simulink model "EV_thermal_charger_2015a_jmaab_Can01"  (R2015a)
settings: Solver=ode3  StartTime=0.0  StopTime=1800  FixedStep=sampling_time  RelTol=1e-3
PreLoadFcn:
  | %run('init_setting.m')
PostLoadFcn:
  | %set_param(gcs, 'SimulationCommand', 'update');
  | %load('save_param/save_P_Charger', 'P_Charger');
  | %load('save_param/save_T_User_set_temp_degC','T_User_set_temp_degC');
  | %load('save_param/save_ENV_PNT_PTTH_Temp_add_degC','ENV_PNT_PTTH_Temp_add_degC');
  | %load('save_param/save_ENV_PNT_CABIN_Temp_add_degC','ENV_PNT_CABIN_Temp_add_degC');
  | %load('save_param/save_ENV_PNT_PHI_Sunlight_W','ENV_PNT_PHI_Sunlight_W');
  | %load('save_param/save_ENV_PNT_Outside_Temp_ini_degC','ENV_PNT_Outside_Temp_ini_degC');
undefined symbols (not defined in the file or in its folder): BK_PNT_Pow_UL, BK_PNT_ReGene_vel_limit_DN_kmph, BK_PNT_ReGene_vel_limit_UP_kmph, BK_PNT_Tau_brake, Brk_LL, Brk_PGain, Brk_UL, BT_PNT_Hi_C_pol_hi_batt, BT_PNT_Hi_Capa_hi_batt_F, BT_PNT_Hi_ocv_SOC_hi_batt_OCV_V_table, BT_PNT_Hi_ocv_SOC_hi_batt_OCV_V_table_x_SOC, BT_PNT_Hi_R_hi_batt_cell, BT_PNT_Hi_R_pol_hi_batt, BT_PNT_Hi_SOC_MAX_hi_batt, BT_PNT_Hi_SOC_MIN_hi_batt, BT_PNT_Hi_SOC_START_hi_batt, BT_PNT_Lo_Capa_lo_batt_F, BT_PNT_Lo_ocv_SOC_lo_batt_OCV_V_table, BT_PNT_Lo_ocv_SOC_lo_batt_OCV_V_table_x_SOC, BT_PNT_Lo_R_lo_batt_ohm, BT_PNT_Lo_SOC_MAX_lo_batt, BT_PNT_Lo_SOC_MIN_lo_batt, BT_PNT_Lo_SOC_START_lo_batt, BTTH_CNT_P_BT_Heater_W, BTTH_CNT_P_BT_Heater_W_x_BTCells_degC, BTTH_CNT_Voltage_BTFan_V, BTTH_CNT_Voltage_BTFan_V_x_BTCells_degC, BTTH_PNT_BT_Heat_Resi_KpW, BTTH_PNT_BT_Heat_Resi_KpW_x_Wind_m3ps, BTTH_PNT_BT_Heater2BTCells_Heat_Resi_KpW, BTTH_PNT_BT_Heater_Heat_Capa_JpK, BTTH_PNT_BTBlock2BTAir_Heat_Resi_KpW, BTTH_PNT_BTBlock_Heat_Capa_JpK, BTTH_PNT_BTCells2BTBlock_Heat_Resi_KpW, BTTH_PNT_BTCells_Heat_Capa_JpK, BTTH_PNT_v_BTFan_Wind_vel_mps, BTTH_PNT_v_BTFan_Wind_vel_mps_x_V_BTFan, CATH_CNT_P_Aircon_W_LL, CATH_CNT_P_Aircon_W_UL, CATH_CNT_P_Gain_Aircon, CATH_CNT_P_Gain_PTC_Heater, CATH_CNT_P_Gain_SeatHT, CATH_CNT_P_PTC_Heater, CATH_CNT_P_PTC_Heater_W_LL, CATH_CNT_P_PTC_Heater_W_UL, CATH_CNT_P_PTC_Heater_x_T_Outside_temp_degC, CATH_CNT_P_SeatHT_W_LL, CATH_CNT_P_SeatHT_W_UL, CATH_CNT_PGain_Temp_blowout, CATH_CNT_T_Aircon_Indoor_degC, CATH_CNT_T_Aircon_Indoor_degC_x_T_blowout_degC, CATH_CNT_T_PTC_Heater_degC_UL, CATH_CNT_T_SeatHT_Temp_degC, CATH_CNT_T_SeatHT_Temp_degC_x_T_blowout_degC, CATH_CNT_V_HVAC_Fan, CATH_CNT_V_HVAC_Fan_x_T_blowout_degC, CATH_CNT_V_RDFan_V, CATH_CNT_V_RDFan_x_P_Aircon_W, CATH_PNT_Air_Convection_Heat_Resi_KpW, CATH_PNT_Air_Convection_Heat_Resi_x_mps ... (+141)
undefined symbols (not defined in the file): ACC_D_Gain, ACC_I_Gain, ACC_P_Gain
libraries: METI_Lib_vehicle_model x52, simulink x35
(part 6 of 6)

== system EV_thermal_charger_2015a_jmaab_Can01/Vehicle/CNT/VCU_CNT/VCU_CNT/trq_MG2_tgtCalc2/回転数上限超過時トルク制限処理 ==
  trq_MG2_tgt : Inport
  w_ROT_motor : Inport  Port=2
  User_Power_req : Inport  Port=3
  Compare To Zero : simulink/Logic and Bit Operations/Compare To Zero  relop=>  OutDataTypeStr=boolean
  Divide_0wari : METI_Lib_vehicle_model/Divide_0wari
  Product : Product
  Subtract2 : Sum  Inputs=+-
  Subtract3 : Sum
  radps2rpm2 : Gain  Gain=radps2rpm
  w_mot_limit : Constant  Value=VCU_CNT_w_mot_limit_rpm
  w_mot_limit1 : Constant  Value=VCU_CNT_w_mot_limit_gain
  flag_overrev : Outport
  trq_MG2_guarded : Outport  Port=2
  wires:
  w_ROT_motor/1 -> radps2rpm2/1
  w_mot_limit/1 -> Subtract2/1
  Subtract2/1 -> Product/1, Compare To Zero/1
  Subtract3/1 -> trq_MG2_guarded/1
  radps2rpm2/1 -> Subtract2/2
  Product/1 -> Divide_0wari/1
  User_Power_req/1 -> Divide_0wari/2
  Compare To Zero/1 -> flag_overrev/1
  trq_MG2_tgt/1 -> Subtract3/2
  Divide_0wari/1 -> Subtract3/1
  w_mot_limit1/1 -> Product/2

== system EV_thermal_charger_2015a_jmaab_Can01/Vehicle/DTTH/DTTH_PNT/DFTH_PNT/DFBlock_Heat_Capacity/degC->K ==
  degC : Inport
  Constant2 : Constant  Value=degC2K
  Sum : Sum  Inputs=++|
  K : Outport
  wires:
  degC/1 -> Sum/2
  Constant2/1 -> Sum/1
  Sum/1 -> K/1

== system EV_thermal_charger_2015a_jmaab_Can01/Vehicle/DTTH/DTTH_PNT/DFTH_PNT/DFOil_Heat_Capacity/degC->K ==
  degC : Inport
  Constant2 : Constant  Value=degC2K
  Sum : Sum  Inputs=++|
  K : Outport
  wires:
  degC/1 -> Sum/2
  Constant2/1 -> Sum/1
  Sum/1 -> K/1

== system EV_thermal_charger_2015a_jmaab_Can01/Vehicle/DTTH/DTTH_PNT/TMTH_PNT/TF_Heat_Capacity/degC->K ==
  degC : Inport
  Constant2 : Constant  Value=degC2K
  Sum : Sum  Inputs=++|
  K : Outport
  wires:
  degC/1 -> Sum/2
  Constant2/1 -> Sum/1
  Sum/1 -> K/1

== system EV_thermal_charger_2015a_jmaab_Can01/Vehicle/DTTH/DTTH_PNT/TMTH_PNT/TMBlock_Heat_Capacity/degC->K ==
  degC : Inport
  Constant2 : Constant  Value=degC2K
  Sum : Sum  Inputs=++|
  K : Outport
  wires:
  degC/1 -> Sum/2
  Constant2/1 -> Sum/1
  Sum/1 -> K/1

== system EV_thermal_charger_2015a_jmaab_Can01/Vehicle/ELTH/ELTH_PNT/INVTH_PNT/INVBlock_Heat_Capacity/degC->K ==
  degC : Inport
  Constant2 : Constant  Value=degC2K
  Sum : Sum  Inputs=++|
  K : Outport
  wires:
  degC/1 -> Sum/2
  Constant2/1 -> Sum/1
  Sum/1 -> K/1

== system EV_thermal_charger_2015a_jmaab_Can01/Vehicle/ELTH/ELTH_PNT/INVTH_PNT/INVTH_Heatsink_Heat_Capacity/degC->K ==
  degC : Inport
  Constant2 : Constant  Value=degC2K
  Sum : Sum  Inputs=++|
  K : Outport
  wires:
  degC/1 -> Sum/2
  Constant2/1 -> Sum/1
  Sum/1 -> K/1

== system EV_thermal_charger_2015a_jmaab_Can01/Vehicle/ELTH/ELTH_PNT/MGTH_PNT/Coil_Heat_Capacity/degC->K ==
  degC : Inport
  Constant2 : Constant  Value=degC2K
  Sum : Sum  Inputs=++|
  K : Outport
  wires:
  degC/1 -> Sum/2
  Constant2/1 -> Sum/1
  Sum/1 -> K/1

== system EV_thermal_charger_2015a_jmaab_Can01/Vehicle/ELTH/ELTH_PNT/MGTH_PNT/MGHousing_Heat_Capacity/degC->K ==
  degC : Inport
  Constant2 : Constant  Value=degC2K
  Sum : Sum  Inputs=++|
  K : Outport
  wires:
  degC/1 -> Sum/2
  Constant2/1 -> Sum/1
  Sum/1 -> K/1

== system EV_thermal_charger_2015a_jmaab_Can01/Vehicle/ELTH/ELTH_PNT/RD_PNT/RDCoolant_Heat_Capacity/degC->K ==
  degC : Inport
  Constant2 : Constant  Value=degC2K
  Sum : Sum  Inputs=++|
  K : Outport
  wires:
  degC/1 -> Sum/2
  Constant2/1 -> Sum/1
  Sum/1 -> K/1

== system EV_thermal_charger_2015a_jmaab_Can01/Vehicle/CATH/CATH_PNT/CABIN/GLASS/CABIN_Glass_Heat_Capacity/degC->K ==
  degC : Inport
  Constant2 : Constant  Value=degC2K
  Sum : Sum  Inputs=++|
  K : Outport
  wires:
  degC/1 -> Sum/2
  Constant2/1 -> Sum/1
  Sum/1 -> K/1

== system EV_thermal_charger_2015a_jmaab_Can01/Vehicle/CATH/CATH_PNT/CABIN/GLASS/CABIN_Glass_Heat_Resistance/Heat_Resistance_Calc ==
  note: ガラス～空気界面の
      | 温度算出
  note: 熱抵抗の合計値算出
  note: 空気の対流による熱伝達の
      | 熱抵抗値を計算
  note: 赤外線輻射による熱伝達の
      | 熱抵抗値を計算
  V_wind_mps : Inport
  S_Heat_Conduction_m2 : Inport  Port=2
  emissivity : Inport  Port=3
  wall_heat_resi : Inport  Port=4
  T_In1_K : Inport  Port=5
  T_Glass_center_K : Inport  Port=6
  Memory : Memory  X0=1e10  InheritSampleTime=on
  R1 : Subsystem
  R2 : Subsystem
  R3 : Subsystem
  Subsystem : Subsystem
  Subsystem1 : Subsystem
  Subsystem2 : Subsystem
      mask Display: image(imread('熱抵抗車外側.jpg'))
  R_total : Outport
  wires:
  Subsystem1/1(T_Glass_surface_K) -> R1/3(T_Glass_surface_K)
  R1/1(R1) -> Subsystem/2(R1)
  R2/1(R2) -> Subsystem/1(R2)
  Memory/1 -> Subsystem1/4(R_total)
  V_wind_mps/1 -> R2/1(V_wind_mps)
  Subsystem/1(R_total) -> R_total/1, Memory/1
  T_In1_K/1 -> Subsystem1/1(T_In1_K), R1/2(T_In1_K)
  T_Glass_center_K/1 -> Subsystem1/2(T_Glass_center_K)
  S_Heat_Conduction_m2/1 -> R3/1(S_Heat_Conduction_m2), R1/4(S_Heat_Conduction_m2), R2/2(S_Heat_Conduction_m2)
  emissivity/1 -> R1/1(emissivity)
  R3/1(R3) -> Subsystem/3(R3), Subsystem1/3(R3)
  wall_heat_resi/1 -> R3/2(wall_heat_resi)

== system EV_thermal_charger_2015a_jmaab_Can01/Vehicle/CATH/CATH_PNT/CABIN/GLASS/CABIN_Glass_Heat_Resistance1/Heat_Resistance_Calc ==
  note: ガラス～空気界面の
      | 温度算出
  note: 熱抵抗の合計値算出
  note: 空気の対流による熱伝達の
      | 熱抵抗値を計算
  note: 赤外線輻射による熱伝達の
      | 熱抵抗値を計算
  V_wind_mps : Inport
  S_Heat_Conduction_m2 : Inport  Port=2
  emissivity : Inport  Port=3
  wall_heat_resi : Inport  Port=4
  T_In1_K : Inport  Port=5
  T_Glass_center_K : Inport  Port=6
  Memory : Memory  X0=1e10  InheritSampleTime=on
  R1 : Subsystem
  R2 : Subsystem
  R3 : Subsystem
  Subsystem : Subsystem
  Subsystem1 : Subsystem
  Subsystem2 : Subsystem
      mask Display: image(imread('熱抵抗車室側.jpg'))
  R_total : Outport
  wires:
  Subsystem1/1(T_Glass_surface_K) -> R1/3(T_Glass_surface_K)
  R1/1(R1) -> Subsystem/2(R1)
  R2/1(R2) -> Subsystem/1(R2)
  Memory/1 -> Subsystem1/4(R_total)
  V_wind_mps/1 -> R2/1(V_wind_mps)
  Subsystem/1(R_total) -> R_total/1, Memory/1
  T_In1_K/1 -> Subsystem1/1(T_In1_K), R1/2(T_In1_K)
  T_Glass_center_K/1 -> Subsystem1/2(T_Glass_center_K)
  S_Heat_Conduction_m2/1 -> R3/1(S_Heat_Conduction_m2), R1/4(S_Heat_Conduction_m2), R2/2(S_Heat_Conduction_m2)
  emissivity/1 -> R1/1(emissivity)
  R3/1(R3) -> Subsystem/3(R3), Subsystem1/3(R3)
  wall_heat_resi/1 -> R3/2(wall_heat_resi)

== system EV_thermal_charger_2015a_jmaab_Can01/Vehicle/CATH/CATH_PNT/CABIN/WALL/CABIN_Wall_Heat_Capacity/degC->K ==
  degC : Inport
  Constant2 : Constant  Value=degC2K
  Sum : Sum  Inputs=++|
  K : Outport
  wires:
  degC/1 -> Sum/2
  Constant2/1 -> Sum/1
  Sum/1 -> K/1

== system EV_thermal_charger_2015a_jmaab_Can01/Vehicle/CATH/CATH_PNT/CABIN/WALL/CABIN_Wall_Heat_Resistance/Heat_Resistance_Calc ==
  note: ガラス～空気界面の
      | 温度算出
  note: 熱抵抗の合計値算出
  note: 空気の対流による熱伝達の
      | 熱抵抗値を計算
  note: 赤外線輻射による熱伝達の
      | 熱抵抗値を計算
  V_wind_mps : Inport
  S_Heat_Conduction_m2 : Inport  Port=2
  emissivity : Inport  Port=3
  wall_heat_resi : Inport  Port=4
  T_In1_K : Inport  Port=5
  T_Glass_center_K : Inport  Port=6
  Memory : Memory  X0=1e10  InheritSampleTime=on
  R1 : Subsystem
  R2 : Subsystem
  R3 : Subsystem
  Subsystem : Subsystem
  Subsystem1 : Subsystem
  Subsystem2 : Subsystem
      mask Display: image(imread('熱抵抗車外側.jpg'))
  R_total : Outport
  wires:
  Subsystem1/1(T_Glass_surface_K) -> R1/3(T_Glass_surface_K)
  R1/1(R1) -> Subsystem/2(R1)
  R2/1(R2) -> Subsystem/1(R2)
  Memory/1 -> Subsystem1/4(R_total)
  V_wind_mps/1 -> R2/1(V_wind_mps)
  Subsystem/1(R_total) -> R_total/1, Memory/1
  T_In1_K/1 -> Subsystem1/1(T_In1_K), R1/2(T_In1_K)
  T_Glass_center_K/1 -> Subsystem1/2(T_Glass_center_K)
  S_Heat_Conduction_m2/1 -> R3/1(S_Heat_Conduction_m2), R1/4(S_Heat_Conduction_m2), R2/2(S_Heat_Conduction_m2)
  emissivity/1 -> R1/1(emissivity)
  R3/1(R3) -> Subsystem/3(R3), Subsystem1/3(R3)
  wall_heat_resi/1 -> R3/2(wall_heat_resi)

== system EV_thermal_charger_2015a_jmaab_Can01/Vehicle/CATH/CATH_PNT/CABIN/WALL/CABIN_Wall_Heat_Resistance1/Heat_Resistance_Calc ==
  note: ガラス～空気界面の
      | 温度算出
  note: 熱抵抗の合計値算出
  note: 空気の対流による熱伝達の
      | 熱抵抗値を計算
  note: 赤外線輻射による熱伝達の
      | 熱抵抗値を計算
  V_wind_mps : Inport
  S_Heat_Conduction_m2 : Inport  Port=2
  emissivity : Inport  Port=3
  wall_heat_resi : Inport  Port=4
  T_In1_K : Inport  Port=5
  T_Glass_center_K : Inport  Port=6
  Memory : Memory  X0=1e10  InheritSampleTime=on
  R1 : Subsystem
  R2 : Subsystem
  R3 : Subsystem
  Subsystem : Subsystem
  Subsystem1 : Subsystem
  Subsystem2 : Subsystem
      mask Display: image(imread('熱抵抗車室側.jpg'))
  R_total : Outport
  wires:
  Subsystem1/1(T_Glass_surface_K) -> R1/3(T_Glass_surface_K)
  R1/1(R1) -> Subsystem/2(R1)
  R2/1(R2) -> Subsystem/1(R2)
  Memory/1 -> Subsystem1/4(R_total)
  V_wind_mps/1 -> R2/1(V_wind_mps)
  Subsystem/1(R_total) -> R_total/1, Memory/1
  T_In1_K/1 -> Subsystem1/1(T_In1_K), R1/2(T_In1_K)
  T_Glass_center_K/1 -> Subsystem1/2(T_Glass_center_K)
  S_Heat_Conduction_m2/1 -> R3/1(S_Heat_Conduction_m2), R1/4(S_Heat_Conduction_m2), R2/2(S_Heat_Conduction_m2)
  emissivity/1 -> R1/1(emissivity)
  R3/1(R3) -> Subsystem/3(R3), Subsystem1/3(R3)
  wall_heat_resi/1 -> R3/2(wall_heat_resi)

== system EV_thermal_charger_2015a_jmaab_Can01/Vehicle/CATH/CATH_PNT/HVAC/Aircon/Aircon_Indoor_Unit_Heat_Capacity1/degC->K ==
  degC : Inport
  Constant2 : Constant  Value=degC2K
  Sum : Sum  Inputs=++|
  K : Outport
  wires:
  degC/1 -> Sum/2
  Constant2/1 -> Sum/1
  Sum/1 -> K/1

== system EV_thermal_charger_2015a_jmaab_Can01/Vehicle/CATH/CATH_PNT/HVAC/Aircon/Aircon_Outdoor_Unit_Heat_Capacity/degC->K ==
  degC : Inport
  Constant2 : Constant  Value=degC2K
  Sum : Sum  Inputs=++|
  K : Outport
  wires:
  degC/1 -> Sum/2
  Constant2/1 -> Sum/1
  Sum/1 -> K/1

== system EV_thermal_charger_2015a_jmaab_Can01/Vehicle/CATH/CATH_PNT/HVAC/PTC_Heater1/PTC_Heater_Heat_Capacity/degC->K ==
  degC : Inport
  Constant2 : Constant  Value=degC2K
  Sum : Sum  Inputs=++|
  K : Outport
  wires:
  degC/1 -> Sum/2
  Constant2/1 -> Sum/1
  Sum/1 -> K/1

== system EV_thermal_charger_2015a_jmaab_Can01/Vehicle/CNT/CHG_CNT/CHG_CNT/Charge_Current_calc/Normal_Charge/Constant_Current_Charge ==
  note: 一定電流充電モード
      | 低SOCでは急速充電器の最大出力電流で制限
      | 高SOCではバッテリ保護のため段階的に電流を減らす
  Maximum_Charge_Current_A : Inport
  SOC_HiBatt : Inport  Port=2
  1-D Lookup Table : Lookup_n-D  NumberOfTableDimensions=1  BreakpointsForDimension1=CHG_CNT_SOC_Adapt_Charge_Current_x_SOC  Table=CHG_CNT_SOC_Adapt_Charge_Current_A  InternalRulePriority=Speed  RndMeth=Simplest  InputSameDT=on
  MinMax : MinMax  Inputs=2
  Current_tgt : Outport
  wires:
  Maximum_Charge_Current_A/1 -> MinMax/1
  SOC_HiBatt/1 -> 1-D Lookup Table/1
  1-D Lookup Table/1 -> MinMax/2
  MinMax/1 -> Current_tgt/1

== system EV_thermal_charger_2015a_jmaab_Can01/Vehicle/CNT/CHG_CNT/CHG_CNT/Charge_Current_calc/Normal_Charge/Constant_Power_Charge ==
  note: 一定出力充電モード
      | 充電器の出力可能な最大電力を出力する
      | 電流値は最大電力÷出力電圧で計算
  Maximum_Charge_Power_W : Inport
  Battery_Voltage_V : Inport  Port=2
  Divide_0wari : METI_Lib_vehicle_model/Divide_0wari
  Current_tgt : Outport
  wires:
  Maximum_Charge_Power_W/1 -> Divide_0wari/1
  Battery_Voltage_V/1 -> Divide_0wari/2
  Divide_0wari/1 -> Current_tgt/1

== system EV_thermal_charger_2015a_jmaab_Can01/Vehicle/CNT/CHG_CNT/CHG_CNT/Charge_Current_calc/Normal_Charge/Constant_Voltage_Charge ==
  note: 一定電圧充電モード
      | 充電の最後の方、高SOCの時に使用する。
      | 出力電圧がバッテリの電圧を超えないように制御
  Maximum_Charge_Current_A : Inport
  Maximum_Charge_Voltage_V : Inport  Port=2
  Maximum_Hi_Batt_SOC : Inport  Port=3
  Battery_Voltage_V : Inport  Port=4
  old_mode : Inport  Port=5
  Add : Sum
  FB : Subsystem
  FF : Subsystem
  MinMax : MinMax  Inputs=2
  MinMax1 : MinMax  Inputs=2
  Subtract : Sum  Inputs=+-
  map_OCV : Lookup  InputValues=BT_PNT_Hi_ocv_SOC_hi_batt_OCV_V_table_x_SOC  Table=BT_PNT_Hi_ocv_SOC_hi_batt_OCV_V_table  LookUpMeth=Interpolation-Use End Values
  Current_tgt : Outport
  wires:
  Maximum_Charge_Voltage_V/1 -> MinMax1/1
  Battery_Voltage_V/1 -> Subtract/2
  Subtract/1 -> FB/1(In1), FF/1(In1)
  FF/1(Out1) -> MinMax/2
  FB/1(Out1) -> Add/2
  Add/1 -> Current_tgt/1
  old_mode/1 -> FB/2(old_mode)
  Maximum_Charge_Current_A/1 -> MinMax/1
  MinMax/1 -> Add/1
  map_OCV/1 -> MinMax1/2
  MinMax1/1 -> Subtract/1
  Maximum_Hi_Batt_SOC/1 -> map_OCV/1

== system EV_thermal_charger_2015a_jmaab_Can01/Vehicle/CATH/CATH_PNT/CABIN/GLASS/CABIN_Glass_Heat_Resistance/Heat_Resistance_Calc/R1 ==
  note: [K/W]
  note: [W/m2K]
  emissivity : Inport
  T_In1_K : Inport  Port=2
  T_Glass_surface_K : Inport  Port=3
  S_Heat_Conduction_m2 : Inport  Port=4
  Add : Sum
  Add1 : Sum
  Constant : Constant  Value=sigma_Stefan_Boltzmann
  Divide : Product  Inputs=/*
  Math Function : Math  Operator=magnitude^2  SaturateOnIntegerOverflow=on
  Math Function1 : Math  Operator=magnitude^2  SaturateOnIntegerOverflow=on
  Product : Product  Inputs=3
  Product1 : Product
  R1 : Outport
  wires:
  T_Glass_surface_K/1 -> Add1/2, Math Function1/1
  Math Function/1 -> Add/1
  Math Function1/1 -> Add/2
  T_In1_K/1 -> Add1/1, Math Function/1
  Add/1 -> Product/2
  Add1/1 -> Product/3
  Product1/1 -> Product/1
  Product/1 -> Divide/1
  Divide/1 -> R1/1
  S_Heat_Conduction_m2/1 -> Divide/2
  Constant/1 -> Product1/1
  emissivity/1 -> Product1/2

== system EV_thermal_charger_2015a_jmaab_Can01/Vehicle/CATH/CATH_PNT/CABIN/GLASS/CABIN_Glass_Heat_Resistance/Heat_Resistance_Calc/R2 ==
  note: [K/W]
  note: [m2K/W]
  note: ユルゲスの実験式による
      | 対流の熱伝達率[W/m2K]を逆数にして
      | 熱抵抗[m2K/W]にしたもの
  V_wind_mps : Inport
  S_Heat_Conduction_m2 : Inport  Port=2
  Abs : Abs
  Air_Convection_Heat_Resi : Lookup_n-D  NumberOfTableDimensions=1  BreakpointsForDimension1=CATH_PNT_Air_Convection_Heat_Resi_x_mps  Table=CATH_PNT_Air_Convection_Heat_Resi_KpW  InternalRulePriority=Speed  RndMeth=Simplest  InputSameDT=on
  Divide : Product  Inputs=*/
  R2 : Outport
  wires:
  V_wind_mps/1 -> Abs/1
  Air_Convection_Heat_Resi/1 -> Divide/1
  Abs/1 -> Air_Convection_Heat_Resi/1
  S_Heat_Conduction_m2/1 -> Divide/2
  Divide/1 -> R2/1

== system EV_thermal_charger_2015a_jmaab_Can01/Vehicle/CATH/CATH_PNT/CABIN/GLASS/CABIN_Glass_Heat_Resistance/Heat_Resistance_Calc/R3 ==
  S_Heat_Conduction_m2 : Inport
  wall_heat_resi : Inport  Port=2
  Divide : Product  Inputs=*/
  R3 : Outport
  wires:
  S_Heat_Conduction_m2/1 -> Divide/2
  wall_heat_resi/1 -> Divide/1
  Divide/1 -> R3/1

== system EV_thermal_charger_2015a_jmaab_Can01/Vehicle/CATH/CATH_PNT/CABIN/GLASS/CABIN_Glass_Heat_Resistance/Heat_Resistance_Calc/Subsystem ==
  note: 直列抵抗部分の
      | 抵抗値計算
      | 単純和
  note: 並列抵抗部分の
      | 抵抗値計算
  R2 : Inport
  R1 : Inport  Port=2
  R3 : Inport  Port=3
  Add : Sum
  Add1 : Sum
  Divide : Product  Inputs=*/
  Product : Product
  R_total : Outport
  wires:
  R1/1 -> Add/1, Product/1
  R2/1 -> Product/2, Add/2
  Product/1 -> Divide/1
  Add/1 -> Divide/2
  Divide/1 -> Add1/1
  Add1/1 -> R_total/1
  R3/1 -> Add1/2

== system EV_thermal_charger_2015a_jmaab_Can01/Vehicle/CATH/CATH_PNT/CABIN/GLASS/CABIN_Glass_Heat_Resistance/Heat_Resistance_Calc/Subsystem1 ==
  T_In1_K : Inport
  T_Glass_center_K : Inport  Port=2
  R3 : Inport  Port=3
  R_total : Inport  Port=4
  Add : Sum
  Divide : Product  Inputs=*/
  Product : Product
  Subtract : Sum  Inputs=-+
  T_Glass_surface_K : Outport
  wires:
  T_Glass_center_K/1 -> Subtract/2
  T_In1_K/1 -> Add/1, Subtract/1
  R3/1 -> Divide/1
  R_total/1 -> Divide/2
  Subtract/1 -> Product/1
  Divide/1 -> Product/2
  Product/1 -> Add/2
  Add/1 -> T_Glass_surface_K/1

== system EV_thermal_charger_2015a_jmaab_Can01/Vehicle/CATH/CATH_PNT/CABIN/GLASS/CABIN_Glass_Heat_Resistance/Heat_Resistance_Calc/Subsystem2 ==

== system EV_thermal_charger_2015a_jmaab_Can01/Vehicle/CATH/CATH_PNT/CABIN/GLASS/CABIN_Glass_Heat_Resistance1/Heat_Resistance_Calc/R1 ==
  note: [K/W]
  note: [W/m2K]
  emissivity : Inport
  T_In1_K : Inport  Port=2
  T_Glass_surface_K : Inport  Port=3
  S_Heat_Conduction_m2 : Inport  Port=4
  Add : Sum
  Add1 : Sum
  Constant : Constant  Value=sigma_Stefan_Boltzmann
  Divide : Product  Inputs=/*
  Math Function : Math  Operator=magnitude^2  SaturateOnIntegerOverflow=on
  Math Function1 : Math  Operator=magnitude^2  SaturateOnIntegerOverflow=on
  Product : Product  Inputs=3
  Product1 : Product
  R1 : Outport
  wires:
  T_Glass_surface_K/1 -> Add1/2, Math Function1/1
  Math Function/1 -> Add/1
  Math Function1/1 -> Add/2
  T_In1_K/1 -> Add1/1, Math Function/1
  Add/1 -> Product/2
  Add1/1 -> Product/3
  Product1/1 -> Product/1
  Product/1 -> Divide/1
  Divide/1 -> R1/1
  S_Heat_Conduction_m2/1 -> Divide/2
  Constant/1 -> Product1/1
  emissivity/1 -> Product1/2

== system EV_thermal_charger_2015a_jmaab_Can01/Vehicle/CATH/CATH_PNT/CABIN/GLASS/CABIN_Glass_Heat_Resistance1/Heat_Resistance_Calc/R2 ==
  note: [K/W]
  note: [m2K/W]
  note: ユルゲスの実験式による
      | 対流の熱伝達率[W/m2K]を逆数にして
      | 熱抵抗[m2K/W]にしたもの
  V_wind_mps : Inport
  S_Heat_Conduction_m2 : Inport  Port=2
  Abs : Abs
  Air_Convection_Heat_Resi : Lookup_n-D  NumberOfTableDimensions=1  BreakpointsForDimension1=CATH_PNT_Air_Convection_Heat_Resi_x_mps  Table=CATH_PNT_Air_Convection_Heat_Resi_KpW  InternalRulePriority=Speed  RndMeth=Simplest  InputSameDT=on
  Divide : Product  Inputs=*/
  R2 : Outport
  wires:
  V_wind_mps/1 -> Abs/1
  Air_Convection_Heat_Resi/1 -> Divide/1
  Abs/1 -> Air_Convection_Heat_Resi/1
  S_Heat_Conduction_m2/1 -> Divide/2
  Divide/1 -> R2/1

== system EV_thermal_charger_2015a_jmaab_Can01/Vehicle/CATH/CATH_PNT/CABIN/GLASS/CABIN_Glass_Heat_Resistance1/Heat_Resistance_Calc/R3 ==
  S_Heat_Conduction_m2 : Inport
  wall_heat_resi : Inport  Port=2
  Divide : Product  Inputs=*/
  R3 : Outport
  wires:
  S_Heat_Conduction_m2/1 -> Divide/2
  wall_heat_resi/1 -> Divide/1
  Divide/1 -> R3/1

== system EV_thermal_charger_2015a_jmaab_Can01/Vehicle/CATH/CATH_PNT/CABIN/GLASS/CABIN_Glass_Heat_Resistance1/Heat_Resistance_Calc/Subsystem ==
  note: 直列抵抗部分の
      | 抵抗値計算
      | 単純和
  note: 並列抵抗部分の
      | 抵抗値計算
  R2 : Inport
  R1 : Inport  Port=2
  R3 : Inport  Port=3
  Add : Sum
  Add1 : Sum
  Divide : Product  Inputs=*/
  Product : Product
  R_total : Outport
  wires:
  R1/1 -> Add/1, Product/1
  R2/1 -> Product/2, Add/2
  Product/1 -> Divide/1
  Add/1 -> Divide/2
  Divide/1 -> Add1/1
  Add1/1 -> R_total/1
  R3/1 -> Add1/2

== system EV_thermal_charger_2015a_jmaab_Can01/Vehicle/CATH/CATH_PNT/CABIN/GLASS/CABIN_Glass_Heat_Resistance1/Heat_Resistance_Calc/Subsystem1 ==
  T_In1_K : Inport
  T_Glass_center_K : Inport  Port=2
  R3 : Inport  Port=3
  R_total : Inport  Port=4
  Add : Sum
  Divide : Product  Inputs=*/
  Product : Product
  Subtract : Sum  Inputs=-+
  T_Glass_surface_K : Outport
  wires:
  T_Glass_center_K/1 -> Subtract/2
  T_In1_K/1 -> Add/1, Subtract/1
  R3/1 -> Divide/1
  R_total/1 -> Divide/2
  Subtract/1 -> Product/1
  Divide/1 -> Product/2
  Product/1 -> Add/2
  Add/1 -> T_Glass_surface_K/1

== system EV_thermal_charger_2015a_jmaab_Can01/Vehicle/CATH/CATH_PNT/CABIN/GLASS/CABIN_Glass_Heat_Resistance1/Heat_Resistance_Calc/Subsystem2 ==

== system EV_thermal_charger_2015a_jmaab_Can01/Vehicle/CATH/CATH_PNT/CABIN/WALL/CABIN_Wall_Heat_Resistance/Heat_Resistance_Calc/R1 ==
  note: [K/W]
  note: [W/m2K]
  emissivity : Inport
  T_In1_K : Inport  Port=2
  T_Glass_surface_K : Inport  Port=3
  S_Heat_Conduction_m2 : Inport  Port=4
  Add : Sum
  Add1 : Sum
  Constant : Constant  Value=sigma_Stefan_Boltzmann
  Divide : Product  Inputs=/*
  Math Function : Math  Operator=magnitude^2  SaturateOnIntegerOverflow=on
  Math Function1 : Math  Operator=magnitude^2  SaturateOnIntegerOverflow=on
  Product : Product  Inputs=3
  Product1 : Product
  R1 : Outport
  wires:
  T_Glass_surface_K/1 -> Add1/2, Math Function1/1
  Math Function/1 -> Add/1
  Math Function1/1 -> Add/2
  T_In1_K/1 -> Add1/1, Math Function/1
  Add/1 -> Product/2
  Add1/1 -> Product/3
  Product1/1 -> Product/1
  Product/1 -> Divide/1
  Divide/1 -> R1/1
  S_Heat_Conduction_m2/1 -> Divide/2
  Constant/1 -> Product1/1
  emissivity/1 -> Product1/2

== system EV_thermal_charger_2015a_jmaab_Can01/Vehicle/CATH/CATH_PNT/CABIN/WALL/CABIN_Wall_Heat_Resistance/Heat_Resistance_Calc/R2 ==
  note: [K/W]
  note: [m2K/W]
  note: ユルゲスの実験式による
      | 対流の熱伝達率[W/m2K]を逆数にして
      | 熱抵抗[m2K/W]にしたもの
  V_wind_mps : Inport
  S_Heat_Conduction_m2 : Inport  Port=2
  Abs : Abs
  Air_Convection_Heat_Resi : Lookup_n-D  NumberOfTableDimensions=1  BreakpointsForDimension1=CATH_PNT_Air_Convection_Heat_Resi_x_mps  Table=CATH_PNT_Air_Convection_Heat_Resi_KpW  InternalRulePriority=Speed  RndMeth=Simplest  InputSameDT=on
  Divide : Product  Inputs=*/
  R2 : Outport
  wires:
  V_wind_mps/1 -> Abs/1
  Air_Convection_Heat_Resi/1 -> Divide/1
  Abs/1 -> Air_Convection_Heat_Resi/1
  S_Heat_Conduction_m2/1 -> Divide/2
  Divide/1 -> R2/1

== system EV_thermal_charger_2015a_jmaab_Can01/Vehicle/CATH/CATH_PNT/CABIN/WALL/CABIN_Wall_Heat_Resistance/Heat_Resistance_Calc/R3 ==
  S_Heat_Conduction_m2 : Inport
  wall_heat_resi : Inport  Port=2
  Divide : Product  Inputs=*/
  R3 : Outport
  wires:
  S_Heat_Conduction_m2/1 -> Divide/2
  wall_heat_resi/1 -> Divide/1
  Divide/1 -> R3/1

== system EV_thermal_charger_2015a_jmaab_Can01/Vehicle/CATH/CATH_PNT/CABIN/WALL/CABIN_Wall_Heat_Resistance/Heat_Resistance_Calc/Subsystem ==
  note: 直列抵抗部分の
      | 抵抗値計算
      | 単純和
  note: 並列抵抗部分の
      | 抵抗値計算
  R2 : Inport
  R1 : Inport  Port=2
  R3 : Inport  Port=3
  Add : Sum
  Add1 : Sum
  Divide : Product  Inputs=*/
  Product : Product
  R_total : Outport
  wires:
  R1/1 -> Add/1, Product/1
  R2/1 -> Product/2, Add/2
  Product/1 -> Divide/1
  Add/1 -> Divide/2
  Divide/1 -> Add1/1
  Add1/1 -> R_total/1
  R3/1 -> Add1/2

== system EV_thermal_charger_2015a_jmaab_Can01/Vehicle/CATH/CATH_PNT/CABIN/WALL/CABIN_Wall_Heat_Resistance/Heat_Resistance_Calc/Subsystem1 ==
  T_In1_K : Inport
  T_Glass_center_K : Inport  Port=2
  R3 : Inport  Port=3
  R_total : Inport  Port=4
  Add : Sum
  Divide : Product  Inputs=*/
  Product : Product
  Subtract : Sum  Inputs=-+
  T_Glass_surface_K : Outport
  wires:
  T_Glass_center_K/1 -> Subtract/2
  T_In1_K/1 -> Add/1, Subtract/1
  R3/1 -> Divide/1
  R_total/1 -> Divide/2
  Subtract/1 -> Product/1
  Divide/1 -> Product/2
  Product/1 -> Add/2
  Add/1 -> T_Glass_surface_K/1

== system EV_thermal_charger_2015a_jmaab_Can01/Vehicle/CATH/CATH_PNT/CABIN/WALL/CABIN_Wall_Heat_Resistance/Heat_Resistance_Calc/Subsystem2 ==

== system EV_thermal_charger_2015a_jmaab_Can01/Vehicle/CATH/CATH_PNT/CABIN/WALL/CABIN_Wall_Heat_Resistance1/Heat_Resistance_Calc/R1 ==
  note: [K/W]
  note: [W/m2K]
  emissivity : Inport
  T_In1_K : Inport  Port=2
  T_Glass_surface_K : Inport  Port=3
  S_Heat_Conduction_m2 : Inport  Port=4
  Add : Sum
  Add1 : Sum
  Constant : Constant  Value=sigma_Stefan_Boltzmann
  Divide : Product  Inputs=/*
  Math Function : Math  Operator=magnitude^2  SaturateOnIntegerOverflow=on
  Math Function1 : Math  Operator=magnitude^2  SaturateOnIntegerOverflow=on
  Product : Product  Inputs=3
  Product1 : Product
  R1 : Outport
  wires:
  T_Glass_surface_K/1 -> Add1/2, Math Function1/1
  Math Function/1 -> Add/1
  Math Function1/1 -> Add/2
  T_In1_K/1 -> Add1/1, Math Function/1
  Add/1 -> Product/2
  Add1/1 -> Product/3
  Product1/1 -> Product/1
  Product/1 -> Divide/1
  Divide/1 -> R1/1
  S_Heat_Conduction_m2/1 -> Divide/2
  Constant/1 -> Product1/1
  emissivity/1 -> Product1/2

== system EV_thermal_charger_2015a_jmaab_Can01/Vehicle/CATH/CATH_PNT/CABIN/WALL/CABIN_Wall_Heat_Resistance1/Heat_Resistance_Calc/R2 ==
  note: [K/W]
  note: [m2K/W]
  note: ユルゲスの実験式による
      | 対流の熱伝達率[W/m2K]を逆数にして
      | 熱抵抗[m2K/W]にしたもの
  V_wind_mps : Inport
  S_Heat_Conduction_m2 : Inport  Port=2
  Abs : Abs
  Air_Convection_Heat_Resi : Lookup_n-D  NumberOfTableDimensions=1  BreakpointsForDimension1=CATH_PNT_Air_Convection_Heat_Resi_x_mps  Table=CATH_PNT_Air_Convection_Heat_Resi_KpW  InternalRulePriority=Speed  RndMeth=Simplest  InputSameDT=on
  Divide : Product  Inputs=*/
  R2 : Outport
  wires:
  V_wind_mps/1 -> Abs/1
  Air_Convection_Heat_Resi/1 -> Divide/1
  Abs/1 -> Air_Convection_Heat_Resi/1
  S_Heat_Conduction_m2/1 -> Divide/2
  Divide/1 -> R2/1

== system EV_thermal_charger_2015a_jmaab_Can01/Vehicle/CATH/CATH_PNT/CABIN/WALL/CABIN_Wall_Heat_Resistance1/Heat_Resistance_Calc/R3 ==
  S_Heat_Conduction_m2 : Inport
  wall_heat_resi : Inport  Port=2
  Divide : Product  Inputs=*/
  R3 : Outport
  wires:
  S_Heat_Conduction_m2/1 -> Divide/2
  wall_heat_resi/1 -> Divide/1
  Divide/1 -> R3/1

== system EV_thermal_charger_2015a_jmaab_Can01/Vehicle/CATH/CATH_PNT/CABIN/WALL/CABIN_Wall_Heat_Resistance1/Heat_Resistance_Calc/Subsystem ==
  note: 直列抵抗部分の
      | 抵抗値計算
      | 単純和
  note: 並列抵抗部分の
      | 抵抗値計算
  R2 : Inport
  R1 : Inport  Port=2
  R3 : Inport  Port=3
  Add : Sum
  Add1 : Sum
  Divide : Product  Inputs=*/
  Product : Product
  R_total : Outport
  wires:
  R1/1 -> Add/1, Product/1
  R2/1 -> Product/2, Add/2
  Product/1 -> Divide/1
  Add/1 -> Divide/2
  Divide/1 -> Add1/1
  Add1/1 -> R_total/1
  R3/1 -> Add1/2

== system EV_thermal_charger_2015a_jmaab_Can01/Vehicle/CATH/CATH_PNT/CABIN/WALL/CABIN_Wall_Heat_Resistance1/Heat_Resistance_Calc/Subsystem1 ==
  T_In1_K : Inport
  T_Glass_center_K : Inport  Port=2
  R3 : Inport  Port=3
  R_total : Inport  Port=4
  Add : Sum
  Divide : Product  Inputs=*/
  Product : Product
  Subtract : Sum  Inputs=-+
  T_Glass_surface_K : Outport
  wires:
  T_Glass_center_K/1 -> Subtract/2
  T_In1_K/1 -> Add/1, Subtract/1
  R3/1 -> Divide/1
  R_total/1 -> Divide/2
  Subtract/1 -> Product/1
  Divide/1 -> Product/2
  Product/1 -> Add/2
  Add/1 -> T_Glass_surface_K/1

== system EV_thermal_charger_2015a_jmaab_Can01/Vehicle/CATH/CATH_PNT/CABIN/WALL/CABIN_Wall_Heat_Resistance1/Heat_Resistance_Calc/Subsystem2 ==

== system EV_thermal_charger_2015a_jmaab_Can01/Vehicle/CNT/CHG_CNT/CHG_CNT/Charge_Current_calc/Normal_Charge/Constant_Voltage_Charge/FB ==
  In1 : Inport
  old_mode : Inport  Port=2
  Constant : Constant  Value=P_Gain_CV_Charge
  Constant1 : Constant  Value=I_Gain_CV_Charge
  Logical Operator : Logic  Operator=NOT  AllPortsSameDT=off  OutDataTypeStr=boolean
  PID Controller : simulink/Continuous/PID Controller  Controller=PI  TimeDomain=Continuous-time  SampleTime=-1  IntegratorMethod=Forward Euler  FilterMethod=Forward Euler  Form=Parallel  UseFilter=on  ControllerParametersSource=external  P=1  I=1  D=0  N=100  InitialConditionSource=internal  InitialConditionForIntegrator=0  InitialConditionForFilter=0  ExternalReset=level  LimitOutput=off  UpperSaturationLimit=inf  LowerSaturationLimit=-inf  LinearizeAsGain=on  AntiWindupMode=none  Kb=1  TrackingMode=off  Kt=1  PParamMin=[]  PParamMax=[]  IParamMin=[]  IParamMax=[]  DParamMin=[]  DParamMax=[]  NParamMin=[]  NParamMax=[]  KbParamMin=[]  KbParamMax=[]  KtParamMin=[]  KtParamMax=[]  POutMin=[]  POutMax=[]  IOutMin=[]  IOutMax=[]  DOutMin=[]  DOutMax=[]  NOutMin=[]  NOutMax=[]  KbOutMin=[]  KbOutMax=[]  KtOutMin=[]  KtOutMax=[]  IntegratorOutMin=[]  IntegratorOutMax=[]  FilterOutMin=[]  FilterOutMax=[]  SumOutMin=[]  SumOutMax=[]  SumI1OutMin=[]  SumI1OutMax=[]  SumI2OutMin=[]  SumI2OutMax=[]  SumI3OutMin=[]  SumI3OutMax=[]  SumDOutMin=[]  SumDOutMax=[]  SaturationOutMin=[]  SaturationOutMax=[]  IntegratorContinuousStateAttributes=''  IntegratorStateMustResolveToSignalObject=off  IntegratorRTWStateStorageClass=Auto  FilterContinuousStateAttributes=''  FilterStateMustResolveToSignalObject=off  FilterRTWStateStorageClass=Auto  DifferentiatorICPrevScaledInput=0  DifferentiatorOutMin=[]  DifferentiatorOutMax=[]
  Out1 : Outport
  wires:
  In1/1 -> PID Controller/1
  PID Controller/1 -> Out1/1
  Constant/1 -> PID Controller/2
  Constant1/1 -> PID Controller/3
  old_mode/1 -> Logical Operator/1
  Logical Operator/1 -> PID Controller/4

== system EV_thermal_charger_2015a_jmaab_Can01/Vehicle/CNT/CHG_CNT/CHG_CNT/Charge_Current_calc/Normal_Charge/Constant_Voltage_Charge/FF ==
  In1 : Inport
  Add : Sum  Inputs=+++
  Constant : Constant  Value=BT_PNT_Hi_R_hi_batt_cell
  Constant1 : Constant  Value=CHG_PNT_Charger_internal_R
  Constant2 : Constant  Value=CHG_PNT_Charger_cable_R
  Divide : Product  Inputs=*/
  Out1 : Outport
  wires:
  In1/1 -> Divide/1
  Divide/1 -> Out1/1
  Add/1 -> Divide/2
  Constant1/1 -> Add/2
  Constant/1 -> Add/1
  Constant2/1 -> Add/3
